simulink model "DisCancelTest"  (R2019a)
settings: Solver=VariableStepAuto  StartTime=0.0  StopTime=20  RelTol=1e-3
settings Model: Creator=Administrator  LastModifiedBy=Administrator

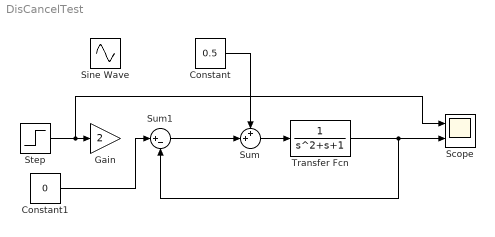
== system DisCancelTest ==
  Constant : Constant  Value=0.5
  Constant1 : Constant  Value=0
  Gain : Gain  Gain=2
  Scope : Scope  NumInputPorts=2
  Sine Wave : Sin  Amplitude=0.2  SampleTime=0
  Step : Step  Time=3  SampleTime=0
  Sum : Sum  Inputs=++|
  Sum1 : Sum  Inputs=|+-
  Transfer Fcn : TransferFcn  Denominator=[1 1 1]
  wires:
  Sum/1 -> Transfer Fcn/1
  Sum1/1 -> Sum/2
  Transfer Fcn/1 -> Sum1/2, Scope/2
  Step/1 -> Scope/1, Gain/1
  Constant1/1 -> Sum1/1
  Constant/1 -> Sum/1
